simulink model "lab4"  (R2019b)
settings: Solver=ode4  StartTime=0.0  StopTime=10.0  RelTol=1e-3
undefined symbols (not defined in the file or in its folder): magnitude
libraries: simulink x2
settings Model: Creator=Michał  LastModifiedBy=Michał

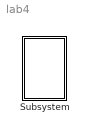
== system lab4 ==
  Subsystem : Subsystem  mask{G=9.81, x=0, y=5, Vx=10, Vy=0, M=200, R=2, Rs=0.05}

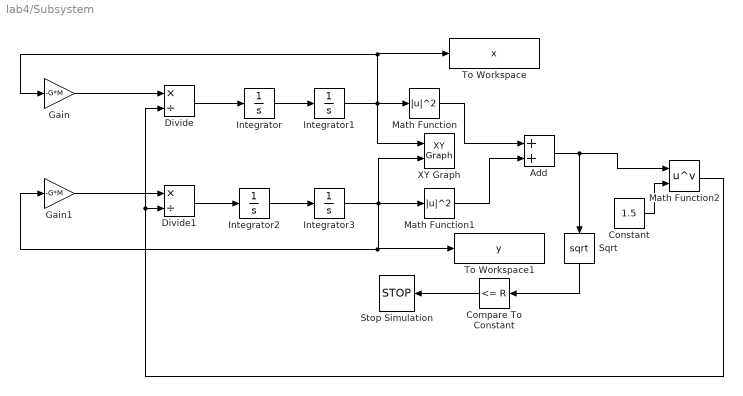
== system lab4/Subsystem ==
  Add : Sum
  Compare To Constant : simulink/Logic and Bit Operations/Compare To Constant  relop=<=  const=R  OutDataTypeStr=boolean
  Constant : Constant  Value=1.5
  Divide : Product  Inputs=*/
  Divide1 : Product  Inputs=*/
  Gain : Gain  Gain=-G*M
  Gain1 : Gain  Gain=-G*M
  Integrator : Integrator  InitialCondition=Vx
  Integrator1 : Integrator  InitialCondition=x
  Integrator2 : Integrator  InitialCondition=Vy
  Integrator3 : Integrator  InitialCondition=y
  Math Function : Math  Operator=magnitude^2  SignedPower=off  SaturateOnIntegerOverflow=on
  Math Function1 : Math  Operator=magnitude^2  SignedPower=off  SaturateOnIntegerOverflow=on
  Math Function2 : Math  Operator=pow  SignedPower=off  SaturateOnIntegerOverflow=on
  Sqrt : Sqrt  SaturateOnIntegerOverflow=on
  Stop Simulation : Stop
  To Workspace : ToWorkspace  VariableName=x  SampleTime=-1
  To Workspace1 : ToWorkspace  VariableName=y  SampleTime=-1
  XY Graph : simulink/Sinks/XY Graph  xmin=-10  xmax=10  ymin=-10  ymax=10  st=2^-7
  wires:
  Add/1 -> Sqrt/1, Math Function2/1
  Gain/1 -> Divide/1
  Integrator2/1 -> Integrator3/1
  Math Function1/1 -> Add/2
  Math Function2/1 -> Divide/2, Divide1/2
  Integrator/1 -> Integrator1/1
  Compare To Constant/1 -> Stop Simulation/1
  Divide1/1 -> Integrator2/1
  Constant/1 -> Math Function2/2
  Divide/1 -> Integrator/1
  Math Function/1 -> Add/1
  Integrator3/1 -> XY Graph/2, To Workspace1/1, Gain1/1, Math Function1/1
  Sqrt/1 -> Compare To Constant/1
  Integrator1/1 -> XY Graph/1, Math Function/1, To Workspace/1, Gain/1
  Gain1/1 -> Divide1/1
